simulink model "debugScope"  (Simulink 8.0)
settings: Solver=FixedStepDiscrete  StartTime=0.0  StopTime=inf  FixedStep=0.01  RelTol=1e-3
libraries: WBCLibrary x2
settings Model: Creator=icub  LastModifiedBy=icub

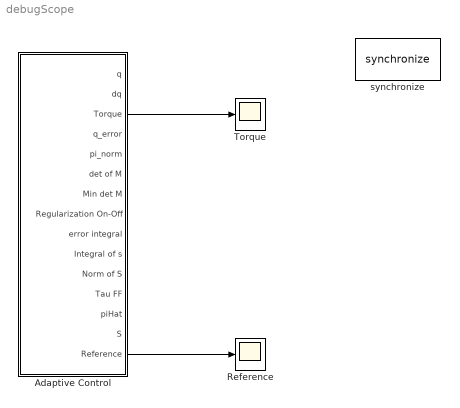
== system debugScope ==
  Adaptive Control : Subsystem  mask{moduleName='adaptiveControl'}
      mask prompts: moduleName "module name"
  Reference : Scope
  Torque : Scope
  synchronize : WBCLibrary/Utilities/synchronize  rate=0.010  scaleFactor=1
  wires:
  Adaptive Control/15(Reference) -> Reference/1
  Adaptive Control/3(Torque) -> Torque/1

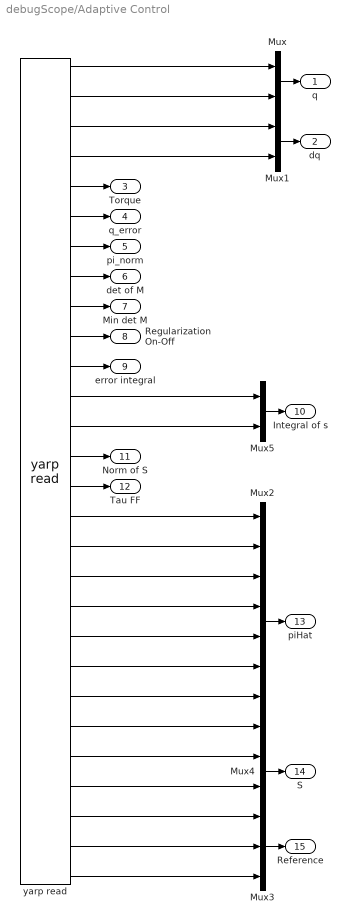
== system debugScope/Adaptive Control ==
  Mux{,1,4..5} (4 alike) : Mux  Inputs=2
  Mux2 : Mux  Inputs=8
  Mux3 : Mux  Inputs=3
  yarp read : WBCLibrary/Utilities/yarp read  from=['/' moduleName '/monitor:o']  to='...'  num=28
  q : Outport
  dq : Outport  Port=2
  Torque : Outport  Port=3
  q_error : Outport  Port=4
  pi_norm : Outport  Port=5
  det of M : Outport  Port=6
  Min det M : Outport  Port=7
  Regularization On-Off : Outport  Port=8
  error integral : Outport  Port=9
  Integral of s : Outport  Port=10
  Norm of S : Outport  Port=11
  Tau FF : Outport  Port=12
  piHat : Outport  Port=13
  S : Outport  Port=14
  Reference : Outport  Port=15
  wires:
  Mux/1 -> q/1
  Mux2/1 -> piHat/1
  yarp read/27 -> Mux3/2
  yarp read/19 -> Mux2/4
  yarp read/23 -> Mux2/8
  yarp read/1 -> Mux/1
  yarp read/18 -> Mux2/3
  yarp read/2 -> Mux/2
  yarp read/24 -> Mux4/1
  yarp read/25 -> Mux4/2
  yarp read/28 -> Mux3/3
  yarp read/26 -> Mux3/1
  yarp read/5 -> Torque/1
  Mux4/1 -> S/1
  yarp read/6 -> q_error/1
  yarp read/8 -> det of M/1
  yarp read/9 -> Min det M/1
  yarp read/7 -> pi_norm/1
  yarp read/10 -> Regularization On-Off/1
  yarp read/15 -> Tau FF/1
  yarp read/11 -> error integral/1
  Mux3/1 -> Reference/1
  Mux1/1 -> dq/1
  yarp read/4 -> Mux1/2
  yarp read/22 -> Mux2/7
  yarp read/3 -> Mux1/1
  yarp read/17 -> Mux2/2
  yarp read/20 -> Mux2/5
  yarp read/16 -> Mux2/1
  yarp read/21 -> Mux2/6
  yarp read/12 -> Mux5/1
  yarp read/13 -> Mux5/2
  Mux5/1 -> Integral of s/1
  yarp read/14 -> Norm of S/1
